simulink model "AEBMIL"  (Simulink 8.2)
settings: Solver=FixedStepDiscrete  StartTime=0.0  StopTime=126  FixedStep=0.005  RelTol=1e-3
PostLoadFcn:
  | , if any(exist('dsrtsu_mdlpostloadfcn', 'file') == [2, 3, 6]), try dsrtsu_mdlpostloadfcn('Execute', bdroot); catch fprintf('Error in PostLoadFcn (dsrtsu_mdlpostloadfcn) for model "%s":\n %s\n', bdroot, lasterr); end, end,
values from neighbouring files (symbols this model uses):
  C_TASK_5MS_S = (	C_TICK_TIME_S      	)    [hcu_local_hdr.m]
  ENUM_GEARPOSN_1ST = uint8(  1  )    [hcu_local_hdr.m]
  ENUM_GEARPOSN_R = uint8(  7  )    [hcu_local_hdr.m]
  FALSE = boolean( 0 )    [hcu_local_hdr.m]
  R_OBJ_Position = single([ii 0 0])    [GridSearch.m]
  R_OBJ_RelAccel = single([0 0 kk])    [GridSearch.m]
  R_OBJ_RelVelocity = single([0 jj 0])    [GridSearch.m]
  TRUE = boolean( 1 )    [hcu_local_hdr.m]
undefined symbols (not defined in the file or in its folder): A_OBJ, AAEB_VehSpd_kph, B_OBJ, C_OBJ, Gamma_OBJ, KAEB_AEBActiveCount_cnt, KAEB_DsblAEBAPPRateThres_pctps, KAEB_DsblAEBSteerRateThres_degps, KAEB_UseMCTTTC_flg, KAEB_VehHoldSpdThres_kph, KOBJ_KalmanFilterCalRate_s, KOBJ_UseCalObjSpd_flg, KOBJ_UseEstObjInfo_flg, KOBJ_VehAccCalRate_s, KOBJ_VehAccFltConst_s, KPTH_ObjPositionYLimit_m, MAEB_AEBTTCThres_s, MAEB_FCWTTCOffset_s, magnitude, MPTH_TurningRadius_m, Q_OBJ, slcm
libraries: simulink x49, hcu_lib x22, dspmtrx3 x3, dspinverses x1
(part 1 of 3)
settings Model: DSRTSU_INTERNAL_RTI_VER=460  DSRTSU_INTERNAL_RTI_TYPE=rti1401  RTICANMMDATA=struct('GeneralSetupData',struct('modelroot','D:\HAITEC\SVN\trunk\ADAS_Softwares\HTDragon\software\sw_development\arch','generalsettings',struct('filesettings',struct('destfolder',struct('Name','RTICANMM_FILES','Check',1),'buildfolder',struct('Name','.','Check',1),'AbsDestfolder',struct('Name','D:\HAITEC\SVN\trunk\ADAS_Softwares\HTDragon\software\sw_development\arch\RTICANMM_FILES'),'AbsBuildfolder',struct('Name','D:\HAITEC\SVN\trunk\ADAS_Softwares\HTDragon\software\sw_development\arch'))),'options',struct('addpaths',1,'rmpaths',1,'addtrcexclusion',logical(1),'cannavigator',struct('checkmonitoring',0),'show_usrtrc',0,'use_usrtrc',0),'advanced',struct('options',[1 1 1 1 1 1 1 1 1 1 1 1 1 1 1 1 1 1 1 1 1 1 1 1 1 1 1 1 1 1 1 1 1 1 1 1 1 1 1 1 1 1 1 1 1 1 1 1 1 1 1 1 1 1 1 1 1 1 1 1 1 1 1 1 1 1 1 1 1 1 1 1 1 1 1 1 1 1 1 1 1 1 1 1 1 1 1 1 1 1 1 1 1 1 1 1 1 1 1 1]),'MPSetup',{{}},'modelname','AEBMIL','block','AEBMIL'))  DSRTSU_INTERNAL_RTIFPGA=50  Creator=14014  LastModifiedBy=14014  BufferReuse=off
settings DataIOCC: SignalLoggingSaveFormat=Dataset
settings OptimizationCC: BlockReduction=off  OptimizeBlockIOStorage=off  BufferReuse=off  ExpressionFolding=off  ExpressionDepthLimit=128  LocalBlockOutputs=off
settings DebuggingCC: FcnCallInpInsideContextMsg=EnableAllAsError  StateNameClashWarn=none
settings HardwareCC: ProdIntDivRoundTo=Zero  ProdEndianess=BigEndian  ProdHWDeviceType=Generic->Custom  TargetIntDivRoundTo=Zero  TargetEndianess=BigEndian  TargetHWDeviceType=Generic->Custom
settings RTWCC: SystemTargetFile=rti1401.tlc  MakeCommand=make_rti  TemplateMakefile=rti1401.tmf  Description=dSPACE DS1401 Hardware Platform  ProcessScript=rti1401_make_rtw_hook
settings STFCustomTargetCC: CodeReplacementLibrary=ANSI_C  ParMdlRefBuildCompliant=on  GeneratePreprocessorConditionals=Disable all  MatFileLogging=on  SystemTargetFile=rti1401.tlc
settings GRTTargetCC: CompOptLevelCompliant=off  ConcurrentExecutionCompliant=off  ExtModeMexFile=noextcomm
settings CustomProperty: DataType=RTWOptions_EnumType_C__Program Files_dSPACE RCPHIL 2015-A_MATLAB_RTI_RTI1401_TLC_rti1401_1InitialSimState  Value=RUN
settings EnumStrPairs: String=RUN

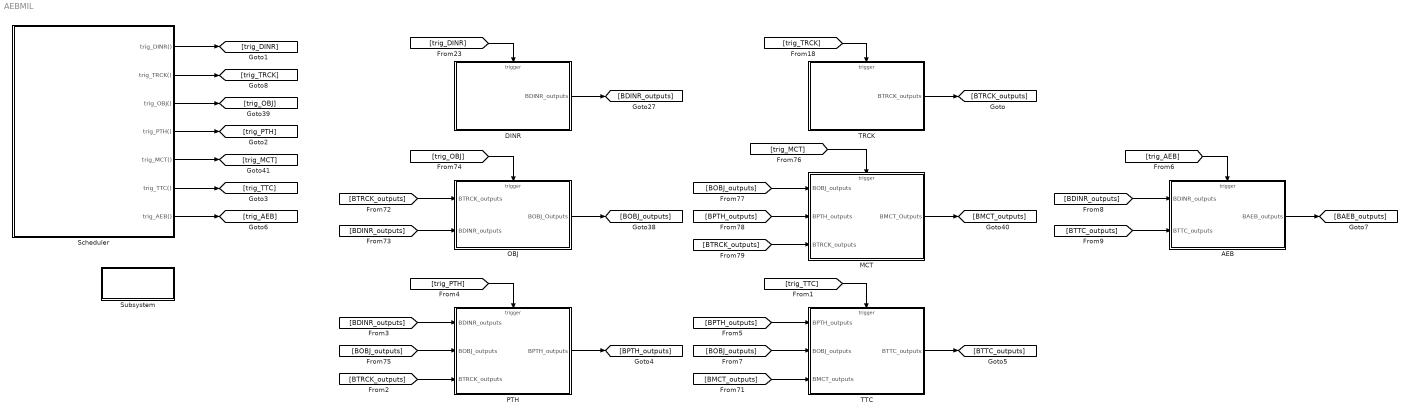
== system AEBMIL ==
  AEB : Subsystem
      settings: RTWSystemCode=Nonreusable function  RTWFcnNameOpts=Use subsystem name  RTWFileNameOpts=Use subsystem name
  DINR : Subsystem
      settings: RTWSystemCode=Nonreusable function  RTWFcnNameOpts=Use subsystem name  RTWFileNameOpts=Use subsystem name
  MCT : Subsystem
      settings: RTWSystemCode=Nonreusable function  RTWFcnNameOpts=Use subsystem name  RTWFileNameOpts=Use subsystem name
  OBJ : Subsystem
      settings: RTWSystemCode=Nonreusable function  RTWFcnNameOpts=Use subsystem name  RTWFileNameOpts=Use subsystem name
  PTH : Subsystem
      settings: RTWSystemCode=Nonreusable function  RTWFcnNameOpts=Use subsystem name  RTWFileNameOpts=Use subsystem name
  Scheduler : Stateflow chart  TreatAsAtomicUnit=on
  Subsystem : Subsystem
      settings: OpenFcn=load AEBMIL_Data.mat;
      mask Display: disp('Double-Click\nTo Load Data')
  TRCK : Subsystem
      settings: RTWSystemCode=Nonreusable function  RTWFcnNameOpts=Use subsystem name  RTWFileNameOpts=Use subsystem name
  TTC : Subsystem
      settings: RTWSystemCode=Nonreusable function  RTWFcnNameOpts=Use subsystem name  RTWFileNameOpts=Use subsystem name
  wires:
  Scheduler/4(trig_PTH()) -> [trig_PTH]
  [BDINR_outputs] -> PTH/1(BDINR_outputs)
  [trig_PTH] -> PTH/Trigger
  PTH/1(BPTH_outputs) -> [BPTH_outputs]
  Scheduler/6(trig_TTC()) -> [trig_TTC]
  [trig_TTC] -> TTC/Trigger
  [BPTH_outputs] -> TTC/1(BPTH_outputs)
  [BOBJ_outputs] -> TTC/2(BOBJ_outputs)
  TTC/1(BTTC_outputs) -> [BTTC_outputs]
  Scheduler/7(trig_AEB()) -> [trig_AEB]
  [trig_AEB] -> AEB/Trigger
  [BDINR_outputs] -> AEB/1(BDINR_outputs)
  [BTTC_outputs] -> AEB/2(BTTC_outputs)
  AEB/1(BAEB_outputs) -> [BAEB_outputs]
  [BMCT_outputs] -> TTC/3(BMCT_outputs)
  [BTRCK_outputs] -> OBJ/1(BTRCK_outputs)
  [BDINR_outputs] -> OBJ/2(BDINR_outputs)
  OBJ/1(BOBJ_Outputs) -> [BOBJ_outputs]
  [trig_OBJ] -> OBJ/Trigger
  Scheduler/3(trig_OBJ()) -> [trig_OBJ]
  [BTRCK_outputs] -> PTH/3(BTRCK_outputs)
  [BOBJ_outputs] -> PTH/2(BOBJ_outputs)
  [trig_MCT] -> MCT/Trigger
  MCT/1(BMCT_Outputs) -> [BMCT_outputs]
  [BOBJ_outputs] -> MCT/1(BOBJ_outputs)
  [BPTH_outputs] -> MCT/2(BPTH_outputs)
  [BTRCK_outputs] -> MCT/3(BTRCK_outputs)
  Scheduler/5(trig_MCT()) -> [trig_MCT]
  [trig_DINR] -> DINR/Trigger
  DINR/1(BDINR_outputs) -> [BDINR_outputs]
  Scheduler/1(trig_DINR()) -> [trig_DINR]
  TRCK/1(BTRCK_outputs) -> [BTRCK_outputs]
  [trig_TRCK] -> TRCK/Trigger
  Scheduler/2(trig_TRCK()) -> [trig_TRCK]

== system AEBMIL/AEB ==
  BDINR_outputs : Inport
  BTTC_outputs : Inport  Port=2  OutDataTypeStr=Bus: BTTC_outputs
  trig_AEB : TriggerPort  TriggerType=function-call
  AEB : Subsystem
  Bus Creator : BusCreator  Inputs=7  OutDataTypeStr=Bus: BAEB_outputs
  Bus Selector : BusSelector  OutputSignals=VTTC_MCTTTC_s,VTTC_Obj1TTCCal_s
  Bus Selector1 : BusSelector  OutputSignals=VDINR_VehSpd_kph,VDINR_SteerAngle_deg,VDINR_SteerAngleValid_flg,VDINR_HWAccelPedalPosn_pct,VDINR_HWAccelPedalPosnValid_flg,VDINR_SeatBeltNOTFasten_flg
  model_info : Subsystem  LoadFcn=slcm LoadBlock;  InitFcn=slcm('UpdateAllCMBlocksInThisModelInit')  mask(CMBlock){InitialSaveTempField=, InitialBlockCM=None, BlockCM=None, Frame=on, SaveTempField=, DisplayStringWithTags=$Id: aeb.mdl 800 2014-08-28 03:32:11Z JuneXmas $, MaskDisplayString=$Id: aeb.mdl 800 2014-08-28 03:32:11Z JuneXmas $, HorizontalTextAlignment=Center, LeftAlignmentValue=0.5, SourceBlockDiagram=AEBMIL, TagMaxNumber=20, CMTag1=, CMTag2=, CMTag3=, CMTag4=, CMTag5=, CMTag6=, CMTag7=, CMTag8=, CMTag9=, CMTag10=, CMTag11=, CMTag12=, CMTag13=, CMTag14=, CMTag15=, CMTag16=, CMTag17=, CMTag18=, CMTag19=, CMTag20=}
      mask help: This block allows revision control information to be displayed within the model.
      settings: CopyFcn=slcm CopyBlock;  DeleteFcn=slcm Cancel;  PostSaveFcn=slcm('UpdateAllCMBlocksInThisModel')  NameChangeFcn=slcm Rename;  OpenFcn=slcm
      mask Display: text(str2num(LeftAlignmentValue), 0.5, MaskDisplayString, 'HorizontalAlignment', HorizontalTextAlignment)
  BAEB_outputs : Outport  OutDataTypeStr=Bus: BAEB_outputs
  wires:
  Bus Selector/2 -> AEB/8(VTTC_Obj1TTCCal_s)  "<VTTC_Obj1TTCCal_s>"
  AEB/7(VAEB_DriverDisable_flg) -> Bus Creator/7
  AEB/6(VAEB_DriverDisableLatch_flg) -> Bus Creator/6
  AEB/5(VAEB_VehHoldReq_flg) -> Bus Creator/5
  AEB/4(VAEB_PreFillReq_flg) -> Bus Creator/4
  AEB/3(VAEB_ForcedIdle_flg) -> Bus Creator/3
  AEB/2(VAEB_FCWActive_flg) -> Bus Creator/2
  AEB/1(VAEB_AEBActive_flg) -> Bus Creator/1
  Bus Creator/1 -> BAEB_outputs/1  "BAEB_outputs"
  BDINR_outputs/1 -> Bus Selector1/1
  Bus Selector1/2 -> AEB/2(VDINR_SteerAngle_deg)  "<VDINR_SteerAngle_deg>"
  Bus Selector1/3 -> AEB/3(VDINR_SteerAngleValid_flg)  "<VDINR_SteerAngleValid_flg>"
  Bus Selector1/4 -> AEB/4(VDINR_HWAccelPedalPosn_pct)  "<VDINR_HWAccelPedalPosn_pct>"
  Bus Selector1/5 -> AEB/5(VDINR_HWAccelPedalPosnValid_flg)  "<VDINR_HWAccelPedalPosnValid_flg>"
  Bus Selector1/6 -> AEB/6(VDINR_SeatBeltNOTFasten_flg)  "<VDINR_SeatBeltNOTFasten_flg>"
  Bus Selector/1 -> AEB/7(VTTC_MCTTTC_s)  "<VTTC_MCTTTC_s>"
  BTTC_outputs/1 -> Bus Selector/1
  Bus Selector1/1 -> AEB/1(VDINR_VehSpd_kph)  "<VDINR_VehSpd_kph>"

== system AEBMIL/DINR ==
  trig_DINR : TriggerPort  TriggerType=function-call
  Bus Creator : BusCreator  Inputs=7
  Cast173 : DataTypeConversion  OutDataTypeStr=boolean  RndMeth=Zero
  Cast202 : DataTypeConversion  OutDataTypeStr=uint8  RndMeth=Zero
  Cast222 : DataTypeConversion  OutDataTypeStr=single  RndMeth=Zero
  Cast259 : DataTypeConversion  OutDataTypeStr=single  RndMeth=Zero
  Cast260 : DataTypeConversion  OutDataTypeStr=boolean  RndMeth=Zero
  Cast89 : DataTypeConversion  OutDataTypeStr=single  RndMeth=Zero
  Cast91 : DataTypeConversion  OutDataTypeStr=boolean  RndMeth=Zero
  Constant : Constant  Value=ENUM_GEARPOSN_1ST
  Constant1 : Constant  Value=TRUE
  Constant2 : Constant  Value=FALSE
  Constant3 : Constant  Value=TRUE
  Constant4 : Constant  Value=single(0)
  From Workspace : FromWorkspace  VariableName=[SimTime VehSpd_kph]
  From Workspace1 : FromWorkspace  VariableName=[SimTime SteerAngle_deg]
  BDINR_outputs : Outport
  wires:
  Constant3/1 -> Cast260/1
  Constant4/1 -> Cast259/1
  Constant2/1 -> Cast173/1
  From Workspace1/1 -> Cast222/1
  Constant1/1 -> Cast91/1
  From Workspace/1 -> Cast89/1
  Constant/1 -> Cast202/1
  Cast260/1 -> Bus Creator/7  "VDINR_HWAccelPedalPosnValid_flg"
  Cast259/1 -> Bus Creator/6  "VDINR_HWAccelPedalPosn_pct"
  Cast173/1 -> Bus Creator/5  "VDINR_SeatBeltNOTFasten_flg"
  Cast202/1 -> Bus Creator/1  "VDINR_NowGearPosn_enum"
  Cast222/1 -> Bus Creator/3  "VDINR_SteerAngle_deg"
  Cast91/1 -> Bus Creator/4  "VDINR_SteerAngleValid_flg"
  Cast89/1 -> Bus Creator/2  "VDINR_VehSpd_kph"
  Bus Creator/1 -> BDINR_outputs/1  "BDINR_outputs"

== system AEBMIL/MCT ==
  BOBJ_outputs : Inport  OutDataTypeStr=Bus: BOBJ_outputs
  BPTH_outputs : Inport  Port=2  OutDataTypeStr=Bus: BPTH_outputs
  BTRCK_outputs : Inport  Port=3  OutDataTypeStr=Bus: BTRCK_outputs
  trig_MCT : TriggerPort  TriggerType=function-call
  Bus Creator : BusCreator  Inputs=5  OutDataTypeStr=Bus: BMCT_outputs
  Bus Selector1 : BusSelector  OutputSignals=VTRCK_Obj1PositionY_m,VTRCK_Obj2PositionY_m,VTRCK_Obj3PositionY_m,VTRCK_Obj4PositionY_m,VTRCK_Obj5PositionY_m
  Bus Selector3 : BusSelector  OutputSignals=VOBJ_Obj1PositionX_m,VOBJ_Obj2PositionX_m,VOBJ_Obj3PositionX_m,VOBJ_Obj4PositionX_m,VOBJ_Obj5PositionX_m,VOBJ_Obj1RelVelocityX_mps,VOBJ_Obj2RelVelocityX_mps,VOBJ_Obj3RelVelocityX_mps,VOBJ_Obj4RelVelocityX_mps,VOBJ_Obj5RelVelocityX_mps,VOBJ_Obj1RelAccX_mps2,VOBJ_Obj2RelAccX_mps2,VOBJ_Obj3RelAccX_mps2,VOBJ_Obj4RelAccX_mps2,VOBJ_Obj5RelAccX_mps2,VOBJ_Obj1Valid_flg,VOBJ_Obj2Valid_flg,VOBJ_Obj3Valid_flg,VOBJ_Obj4Valid_flg,VOBJ_Obj5Valid_flg
  Bus Selector5 : BusSelector  OutputSignals=VPTH_HostPathYOfstWRTObj1_m,VPTH_HostPathYOfstWRTObj2_m,VPTH_HostPathYOfstWRTObj3_m,VPTH_HostPathYOfstWRTObj4_m,VPTH_HostPathYOfstWRTObj5_m,VPTH_Obj1InPath_flg,VPTH_Obj2InPath_flg,VPTH_Obj3InPath_flg,VPTH_Obj4InPath_flg,VPTH_Obj5InPath_flg
  MCT : Subsystem
  model_info : Subsystem  LoadFcn=slcm LoadBlock;  InitFcn=slcm('UpdateAllCMBlocksInThisModelInit')  mask(CMBlock){InitialSaveTempField=, InitialBlockCM=None, BlockCM=None, Frame=on, SaveTempField=, DisplayStringWithTags=$Id: ttc.mdl 800 2014-08-28 03:32:11Z JuneXmas $, MaskDisplayString=$Id: ttc.mdl 800 2014-08-28 03:32:11Z JuneXmas $, HorizontalTextAlignment=Center, LeftAlignmentValue=0.5, SourceBlockDiagram=AEBMIL, TagMaxNumber=20, CMTag1=, CMTag2=, CMTag3=, CMTag4=, CMTag5=, CMTag6=, CMTag7=, CMTag8=, CMTag9=, CMTag10=, CMTag11=, CMTag12=, CMTag13=, CMTag14=, CMTag15=, CMTag16=, CMTag17=, CMTag18=, CMTag19=, CMTag20=}
      mask help: This block allows revision control information to be displayed within the model.
      settings: CopyFcn=slcm CopyBlock;  DeleteFcn=slcm Cancel;  PostSaveFcn=slcm('UpdateAllCMBlocksInThisModel')  NameChangeFcn=slcm Rename;  OpenFcn=slcm
      mask Display: text(str2num(LeftAlignmentValue), 0.5, MaskDisplayString, 'HorizontalAlignment', HorizontalTextAlignment)
  BMCT_Outputs : Outport  OutDataTypeStr=Bus: BMCT_outputs
  wires:
  MCT/5(VMCT_MCTInPath_flg) -> Bus Creator/5
  Bus Selector5/6 -> MCT/31(VPTH_Obj1InPath_flg)  "<VPTH_Obj1InPath_flg>"
  Bus Selector5/7 -> MCT/32(VPTH_Obj2InPath_flg)  "<VPTH_Obj2InPath_flg>"
  Bus Selector5/8 -> MCT/33(VPTH_Obj3InPath_flg)  "<VPTH_Obj3InPath_flg>"
  Bus Selector5/9 -> MCT/34(VPTH_Obj4InPath_flg)  "<VPTH_Obj4InPath_flg>"
  Bus Selector5/10 -> MCT/35(VPTH_Obj5InPath_flg)  "<VPTH_Obj5InPath_flg>"
  MCT/4(VMCT_MCTValid_flg) -> Bus Creator/4
  MCT/3(VMCT_MCTRelAccX_mps2) -> Bus Creator/3
  MCT/2(VMCT_MCTRelVelocityX_mps) -> Bus Creator/2
  MCT/1(VMCT_MCTPositionX_m) -> Bus Creator/1
  Bus Selector5/5 -> MCT/30(VPTH_HostPathYOfstWRTObj5_m)  "<VPTH_HostPathYOfstWRTObj5_m>"
  Bus Selector5/4 -> MCT/29(VPTH_HostPathYOfstWRTObj4_m)  "<VPTH_HostPathYOfstWRTObj4_m>"
  Bus Selector5/3 -> MCT/28(VPTH_HostPathYOfstWRTObj3_m)  "<VPTH_HostPathYOfstWRTObj3_m>"
  Bus Selector5/2 -> MCT/27(VPTH_HostPathYOfstWRTObj2_m)  "<VPTH_HostPathYOfstWRTObj2_m>"
  Bus Selector5/1 -> MCT/26(VPTH_HostPathYOfstWRTObj1_m)  "<VPTH_HostPathYOfstWRTObj1_m>"
  Bus Selector1/5 -> MCT/25(VTRCK_Obj5PositionY_m)  "<VTRCK_Obj5PositionY_m>"
  Bus Selector1/4 -> MCT/24(VTRCK_Obj4PositionY_m)  "<VTRCK_Obj4PositionY_m>"
  Bus Selector1/3 -> MCT/23(VTRCK_Obj3PositionY_m)  "<VTRCK_Obj3PositionY_m>"
  Bus Selector1/2 -> MCT/22(VTRCK_Obj2PositionY_m)  "<VTRCK_Obj2PositionY_m>"
  Bus Selector1/1 -> MCT/21(VTRCK_Obj1PositionY_m)  "<VTRCK_Obj1PositionY_m>"
  BTRCK_outputs/1 -> Bus Selector1/1
  Bus Selector3/20 -> MCT/20(VOBJ_Obj5Valid_flg)  "<VOBJ_Obj5Valid_flg>"
  Bus Selector3/19 -> MCT/19(VOBJ_Obj4Valid_flg)  "<VOBJ_Obj4Valid_flg>"
  Bus Selector3/18 -> MCT/18(VOBJ_Obj3Valid_flg)  "<VOBJ_Obj3Valid_flg>"
  Bus Selector3/17 -> MCT/17(VOBJ_Obj2Valid_flg)  "<VOBJ_Obj2Valid_flg>"
  Bus Selector3/16 -> MCT/16(VOBJ_Obj1Valid_flg)  "<VOBJ_Obj1Valid_flg>"
  Bus Selector3/15 -> MCT/15(VOBJ_Obj5RelAccX_mps2)  "<VOBJ_Obj5RelAccX_mps2>"
  Bus Selector3/14 -> MCT/14(VOBJ_Obj4RelAccX_mps2)  "<VOBJ_Obj4RelAccX_mps2>"
  Bus Selector3/13 -> MCT/13(VOBJ_Obj3RelAccX_mps2)  "<VOBJ_Obj3RelAccX_mps2>"
  Bus Selector3/12 -> MCT/12(VOBJ_Obj2RelAccX_mps2)  "<VOBJ_Obj2RelAccX_mps2>"
  Bus Selector3/11 -> MCT/11(VOBJ_Obj1RelAccX_mps2)  "<VOBJ_Obj1RelAccX_mps2>"
  Bus Selector3/10 -> MCT/10(VOBJ_Obj5RelVelocityX_mps)  "<VOBJ_Obj5RelVelocityX_mps>"
  Bus Selector3/9 -> MCT/9(VOBJ_Obj4RelVelocityX_mps)  "<VOBJ_Obj4RelVelocityX_mps>"
  Bus Selector3/8 -> MCT/8(VOBJ_Obj3RelVelocityX_mps)  "<VOBJ_Obj3RelVelocityX_mps>"
  Bus Selector3/7 -> MCT/7(VOBJ_Obj2RelVelocityX_mps)  "<VOBJ_Obj2RelVelocityX_mps>"
  Bus Selector3/6 -> MCT/6(VOBJ_Obj1RelVelocityX_mps)  "<VOBJ_Obj1RelVelocityX_mps>"
  Bus Selector3/5 -> MCT/5(VObj_Obj5PositionX_m)  "<VOBJ_Obj5PositionX_m>"
  Bus Selector3/1 -> MCT/1(VOBJ_Obj1PositionX_m)  "<VOBJ_Obj1PositionX_m>"
  Bus Selector3/4 -> MCT/4(VOBJ_Obj4PositionX_m)  "<VOBJ_Obj4PositionX_m>"
  Bus Selector3/2 -> MCT/2(VOBJ_Obj2PositionX_m)  "<VOBJ_Obj2PositionX_m>"
  Bus Selector3/3 -> MCT/3(VOBJ_Obj3PositionX_m)  "<VOBJ_Obj3PositionX_m>"
  BPTH_outputs/1 -> Bus Selector5/1
  BOBJ_outputs/1 -> Bus Selector3/1
  Bus Creator/1 -> BMCT_Outputs/1  "BMCT_outputs"

== system AEBMIL/OBJ ==
  BTRCK_outputs : Inport  OutDataTypeStr=Bus: BTRCK_outputs
  BDINR_outputs : Inport  Port=2
  trig_OBJ : TriggerPort  TriggerType=function-call
  Bus Creator : BusCreator  Inputs=20  OutDataTypeStr=Bus: BOBJ_outputs
  Bus Selector3 : BusSelector  OutputSignals=VTRCK_Obj1PositionX_m,VTRCK_Obj1RelVelocityX_mps,VTRCK_Obj1Valid_flg,VTRCK_Obj1ConfidLevel_enum,VTRCK_Obj2PositionX_m,VTRCK_Obj2RelVelocityX_mps,VTRCK_Obj2Valid_flg,VTRCK_Obj2ConfidLevel_enum,VTRCK_Obj3PositionX_m,VTRCK_Obj3RelVelocityX_mps,VTRCK_Obj3Valid_flg,VTRCK_Obj3ConfidLevel_enum,VTRCK_Obj4PositionX_m,VTRCK_Obj4RelVelocityX_mps,VTRCK_Obj4Valid_flg,VTRCK_Obj4ConfidLevel_enum,VTRCK_Obj5PositionX_m,VTRCK_Obj5RelVelocityX_mps,VTRCK_Obj5Valid_flg,VTRCK_Obj5ConfidLevel_enum
  Bus Selector5 : BusSelector  OutputSignals=VDINR_VehSpd_kph,VDINR_NowGearPosn_enum
  OBJ : Subsystem
  model_info : Subsystem  LoadFcn=slcm LoadBlock;  InitFcn=slcm('UpdateAllCMBlocksInThisModelInit')  mask(CMBlock){InitialSaveTempField=, InitialBlockCM=None, BlockCM=None, Frame=on, SaveTempField=, DisplayStringWithTags=$Id: ttc.mdl 800 2014-08-28 03:32:11Z JuneXmas $, MaskDisplayString=$Id: ttc.mdl 800 2014-08-28 03:32:11Z JuneXmas $, HorizontalTextAlignment=Center, LeftAlignmentValue=0.5, SourceBlockDiagram=AEBMIL, TagMaxNumber=20, CMTag1=, CMTag2=, CMTag3=, CMTag4=, CMTag5=, CMTag6=, CMTag7=, CMTag8=, CMTag9=, CMTag10=, CMTag11=, CMTag12=, CMTag13=, CMTag14=, CMTag15=, CMTag16=, CMTag17=, CMTag18=, CMTag19=, CMTag20=}
      mask help: This block allows revision control information to be displayed within the model.
      settings: CopyFcn=slcm CopyBlock;  DeleteFcn=slcm Cancel;  PostSaveFcn=slcm('UpdateAllCMBlocksInThisModel')  NameChangeFcn=slcm Rename;  OpenFcn=slcm
      mask Display: text(str2num(LeftAlignmentValue), 0.5, MaskDisplayString, 'HorizontalAlignment', HorizontalTextAlignment)
  BOBJ_Outputs : Outport  OutDataTypeStr=Bus: BOBJ_outputs
  wires:
  Bus Creator/1 -> BOBJ_Outputs/1  "BOBJ_outputs"
  BTRCK_outputs/1 -> Bus Selector3/1
  Bus Selector3/14 -> OBJ/14(VTRCK_Obj4RelVelocityX_mps)  "<VTRCK_Obj4RelVelocityX_mps>"
  Bus Selector3/10 -> OBJ/10(VTRCK_Obj3RelVelocityX_mps)  "<VTRCK_Obj3RelVelocityX_mps>"
  Bus Selector3/9 -> OBJ/9(VTRCK_Obj3PositionX_m)  "<VTRCK_Obj3PositionX_m>"
  Bus Selector3/2 -> OBJ/2(VTRCK_Obj1RelVelocityX_mps)  "<VTRCK_Obj1RelVelocityX_mps>"
  Bus Selector3/6 -> OBJ/6(VTRCK_Obj2RelVelocityX_mps)  "<VTRCK_Obj2RelVelocityX_mps>"
  Bus Selector3/18 -> OBJ/18(VTRCK_Obj5RelVelocityX_mps)  "<VTRCK_Obj5RelVelocityX_mps>"
  Bus Selector3/1 -> OBJ/1(VTRCK_Obj1PositionX_m)  "<VTRCK_Obj1PositionX_m>"
  Bus Selector3/5 -> OBJ/5(VTRCK_Obj2PositionX_m)  "<VTRCK_Obj2PositionX_m>"
  Bus Selector3/13 -> OBJ/13(VTRCK_Obj4PositionX_m)  "<VTRCK_Obj4PositionX_m>"
  Bus Selector3/17 -> OBJ/17(VTRCK_Obj5PositionX_m)  "<VTRCK_Obj5PositionX_m>"
  Bus Selector5/1 -> OBJ/21(VDINR_VehSpd_kph)  "<VDINR_VehSpd_kph>"
  BDINR_outputs/1 -> Bus Selector5/1
  Bus Selector3/3 -> OBJ/3(VTRCK_Obj1Valid_flg)  "<VTRCK_Obj1Valid_flg>"
  Bus Selector3/7 -> OBJ/7(VTRCK_Obj2Valid_flg)  "<VTRCK_Obj2Valid_flg>"
  Bus Selector3/11 -> OBJ/11(VTRCK_Obj3Valid_flg)  "<VTRCK_Obj3Valid_flg>"
  Bus Selector3/15 -> OBJ/15(VTRCK_Obj4Valid_flg)  "<VTRCK_Obj4Valid_flg>"
  Bus Selector3/19 -> OBJ/19(VTRCK_Obj5Valid_flg)  "<VTRCK_Obj5Valid_flg>"
  OBJ/1(VOBJ_Obj1PositionX_m) -> Bus Creator/1
  OBJ/2(VOBJ_Obj1RelVelocityX_mps) -> Bus Creator/2
  OBJ/3(VOBJ_Obj1RelAccX_mps2) -> Bus Creator/3
  OBJ/4(VOBJ_Obj1Valid_flg) -> Bus Creator/4
  OBJ/5(VOBJ_Obj2PositionX_m) -> Bus Creator/5
  OBJ/6(VOBJ_Obj2RelVelocityX_mps) -> Bus Creator/6
  OBJ/7(VOBJ_Obj2RelAccX_mps2) -> Bus Creator/7
  OBJ/8(VOBJ_Obj2Valid_flg) -> Bus Creator/8
  OBJ/9(VOBJ_Obj3PositionX_m) -> Bus Creator/9
  OBJ/10(VOBJ_Obj3RelVelocityX_mps) -> Bus Creator/10
  OBJ/11(VOBJ_Obj3RelAccX_mps2) -> Bus Creator/11
  OBJ/12(VOBJ_Obj3Valid_flg) -> Bus Creator/12
  OBJ/13(VOBJ_Obj4PositionX_m) -> Bus Creator/13
  OBJ/14(VOBJ_Obj4RelVelocityX_mps) -> Bus Creator/14
  OBJ/15(VOBJ_Obj4RelAccX_mps2) -> Bus Creator/15
  OBJ/16(VOBJ_Obj4Valid_flg) -> Bus Creator/16
  OBJ/17(VOBJ_Obj5PositionX_m) -> Bus Creator/17
  OBJ/18(VOBJ_Obj5RelVelocityX_mps) -> Bus Creator/18
  OBJ/19(VOBJ_Obj5RelAccX_mps2) -> Bus Creator/19
  OBJ/20(VOBJ_Obj5Valid_flg) -> Bus Creator/20
  Bus Selector5/2 -> OBJ/22(VDINR_NowGearPosn_enum)  "<VDINR_NowGearPosn_enum>"
  Bus Selector3/4 -> OBJ/4(VTRCK_Obj1ConfidLevel_enum)  "<VTRCK_Obj1ConfidLevel_enum>"
  Bus Selector3/8 -> OBJ/8(VTRCK_Obj2ConfidLevel_enum)  "<VTRCK_Obj2ConfidLevel_enum>"
  Bus Selector3/12 -> OBJ/12(VTRCK_Obj3ConfidLevel_enum)  "<VTRCK_Obj3ConfidLevel_enum>"
  Bus Selector3/16 -> OBJ/16(VTRCK_Obj4ConfidLevel_enum)  "<VTRCK_Obj4ConfidLevel_enum>"
  Bus Selector3/20 -> OBJ/20(VTRCK_Obj5ConfidLevel_enum)  "<VTRCK_Obj5ConfidLevel_enum>"

== system AEBMIL/PTH ==
  BDINR_outputs : Inport
  BOBJ_outputs : Inport  Port=2  OutDataTypeStr=Bus: BOBJ_outputs
  BTRCK_outputs : Inport  Port=3  OutDataTypeStr=Bus: BTRCK_outputs
  trig_PTH : TriggerPort  TriggerType=function-call
  Bus Creator : BusCreator  Inputs=10  OutDataTypeStr=Bus: BPTH_outputs
  Bus Selector : BusSelector  OutputSignals=VDINR_VehSpd_kph,VDINR_SteerAngle_deg,VDINR_SteerAngleValid_flg
  Bus Selector1 : BusSelector  OutputSignals=VTRCK_Obj1PositionY_m,VTRCK_Obj2PositionY_m,VTRCK_Obj3PositionY_m,VTRCK_Obj4PositionY_m,VTRCK_Obj5PositionY_m
  Bus Selector2 : BusSelector  OutputSignals=VOBJ_Obj1PositionX_m,VOBJ_Obj2PositionX_m,VOBJ_Obj3PositionX_m,VOBJ_Obj4PositionX_m,VOBJ_Obj5PositionX_m,VOBJ_Obj1Valid_flg,VOBJ_Obj2Valid_flg,VOBJ_Obj3Valid_flg,VOBJ_Obj4Valid_flg,VOBJ_Obj5Valid_flg
  PathEstimation : Subsystem
  model_info : Subsystem  LoadFcn=slcm LoadBlock;  InitFcn=slcm('UpdateAllCMBlocksInThisModelInit')  mask(CMBlock){InitialSaveTempField=, InitialBlockCM=None, BlockCM=None, Frame=on, SaveTempField=, DisplayStringWithTags=$Id: pth.mdl 800 2014-08-28 03:32:11Z JuneXmas $, MaskDisplayString=$Id: pth.mdl 800 2014-08-28 03:32:11Z JuneXmas $, HorizontalTextAlignment=Center, LeftAlignmentValue=0.5, SourceBlockDiagram=AEBMIL, TagMaxNumber=20, CMTag1=, CMTag2=, CMTag3=, CMTag4=, CMTag5=, CMTag6=, CMTag7=, CMTag8=, CMTag9=, CMTag10=, CMTag11=, CMTag12=, CMTag13=, CMTag14=, CMTag15=, CMTag16=, CMTag17=, CMTag18=, CMTag19=, CMTag20=}
      mask help: This block allows revision control information to be displayed within the model.
      settings: CopyFcn=slcm CopyBlock;  DeleteFcn=slcm Cancel;  PostSaveFcn=slcm('UpdateAllCMBlocksInThisModel')  NameChangeFcn=slcm Rename;  OpenFcn=slcm
      mask Display: text(str2num(LeftAlignmentValue), 0.5, MaskDisplayString, 'HorizontalAlignment', HorizontalTextAlignment)
  BPTH_outputs : Outport  OutDataTypeStr=Bus: BPTH_outputs
  wires:
  PathEstimation/10(VPTH_HostPathYOfstWRTObj5_m) -> Bus Creator/10
  PathEstimation/9(VPTH_HostPathYOfstWRTObj4_m) -> Bus Creator/9
  PathEstimation/8(VPTH_HostPathYOfstWRTObj3_m) -> Bus Creator/8
  PathEstimation/7(VPTH_HostPathYOfstWRTObj2_m) -> Bus Creator/7
  PathEstimation/6(VPTH_HostPathYOfstWRTObj1_m) -> Bus Creator/6
  Bus Selector2/7 -> PathEstimation/10(VOBJ_Obj2Valid_flg)  "<VOBJ_Obj2Valid_flg>"
  Bus Selector2/8 -> PathEstimation/11(VOBJ_Obj3Valid_flg)  "<VOBJ_Obj3Valid_flg>"
  Bus Selector2/6 -> PathEstimation/9(VOBJ_Obj1Valid_flg)  "<VOBJ_Obj1Valid_flg>"
  Bus Selector2/10 -> PathEstimation/13(VOBJ_Obj5Valid_flg)  "<VOBJ_Obj5Valid_flg>"
  Bus Selector2/9 -> PathEstimation/12(VOBJ_Obj4Valid_flg)  "<VOBJ_Obj4Valid_flg>"
  Bus Selector2/4 -> PathEstimation/7(VOBJ_Obj4PositionX_m)  "<VOBJ_Obj4PositionX_m>"
  Bus Selector2/2 -> PathEstimation/5(VOBJ_Obj2PositionX_m)  "<VOBJ_Obj2PositionX_m>"
  Bus Selector2/5 -> PathEstimation/8(VOBJ_Obj5PositionX_m)  "<VOBJ_Obj5PositionX_m>"
  Bus Selector2/1 -> PathEstimation/4(VOBJ_Obj1PositionX_m)  "<VOBJ_Obj1PositionX_m>"
  Bus Selector2/3 -> PathEstimation/6(VOBJ_Obj3PositionX_m)  "<VOBJ_Obj3PositionX_m>"
  BOBJ_outputs/1 -> Bus Selector2/1
  PathEstimation/4(VPTH_Obj4InPath_flg) -> Bus Creator/4
  PathEstimation/5(VPTH_Obj5InPath_flg) -> Bus Creator/5
  PathEstimation/2(VPTH_Obj2InPath_flg) -> Bus Creator/2
  PathEstimation/1(VPTH_Obj1InPath_flg) -> Bus Creator/1
  PathEstimation/3(VPTH_Obj3InPath_flg) -> Bus Creator/3
  Bus Selector1/5 -> PathEstimation/18(VTRCK_Obj5PositionY_m)  "<VTRCK_Obj5PositionY_m>"
  Bus Selector1/4 -> PathEstimation/17(VTRCK_Obj4PositionY_m)  "<VTRCK_Obj4PositionY_m>"
  Bus Selector1/3 -> PathEstimation/16(VTRCK_Obj3PositionY_m)  "<VTRCK_Obj3PositionY_m>"
  Bus Selector1/2 -> PathEstimation/15(VTRCK_Obj2PositionY_m)  "<VTRCK_Obj2PositionY_m>"
  Bus Selector1/1 -> PathEstimation/14(VTRCK_Obj1PositionY_m)  "<VTRCK_Obj1PositionY_m>"
  BDINR_outputs/1 -> Bus Selector/1
  Bus Creator/1 -> BPTH_outputs/1  "BPTH_outputs"
  Bus Selector/2 -> PathEstimation/2(VDINR_SteerAngle_deg)  "<VDINR_SteerAngle_deg>"
  BTRCK_outputs/1 -> Bus Selector1/1
  Bus Selector/3 -> PathEstimation/3(VDINR_SteerAngleValid_flg)  "<VDINR_SteerAngleValid_flg>"
  Bus Selector/1 -> PathEstimation/1(VDINR_VehSpd_kph)  "<VDINR_VehSpd_kph>"

== system AEBMIL/Subsystem ==

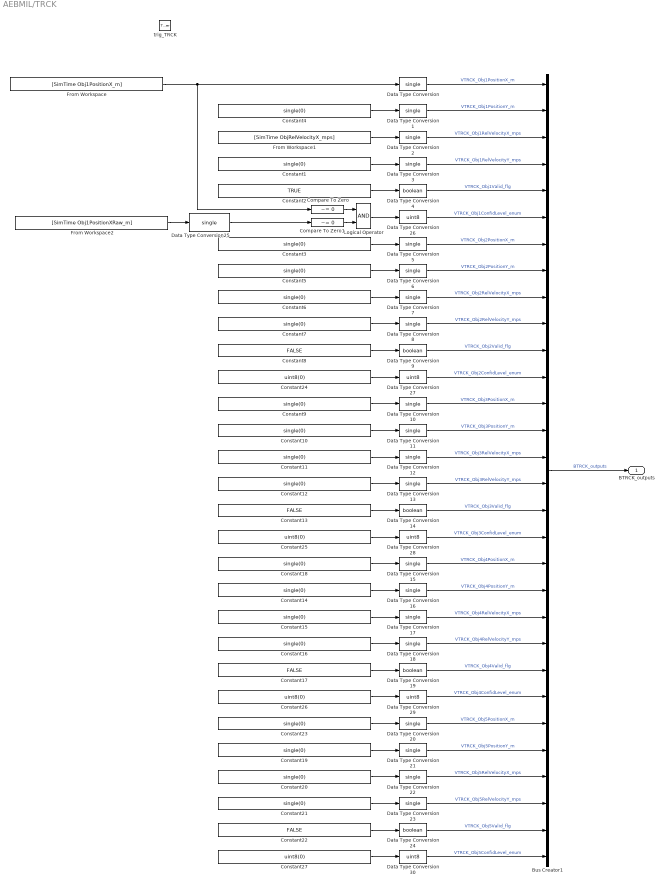
== system AEBMIL/TRCK ==
  trig_TRCK : TriggerPort  TriggerType=function-call
  Bus Creator1 : BusCreator  Inputs=30  OutDataTypeStr=Bus: BTRCK_outputs
  Compare To Zero : simulink/Logic and Bit Operations/Compare To Zero  relop=~=  OutDataTypeStr=boolean
  Compare To Zero1 : simulink/Logic and Bit Operations/Compare To Zero  relop=~=  OutDataTypeStr=boolean
  Constant{1,3..7,9..12,14..16,18..21,23} (18 alike) : Constant  Value=single(0)
  Constant{8,13,17,22} (4 alike) : Constant  Value=FALSE
  Constant2 : Constant  Value=TRUE
  Constant{24..27} (4 alike) : Constant  Value=uint8(0)
  Data Type Conversion{,1..3,5..8,10..13,15..18,20..23,25} (21 alike) : DataTypeConversion  OutDataTypeStr=single
  Data Type Conversion{4,9,14,19,24} (5 alike) : DataTypeConversion  OutDataTypeStr=boolean
  Data Type Conversion{26..30} (5 alike) : DataTypeConversion  OutDataTypeStr=uint8
  From Workspace : FromWorkspace  VariableName=[SimTime Obj1PositionX_m]  Interpolate=off  OutputAfterFinalValue=Setting to zero
  From Workspace1 : FromWorkspace  VariableName=[SimTime ObjRelVelocityX_mps]  Interpolate=off  OutputAfterFinalValue=Setting to zero
  From Workspace2 : FromWorkspace  VariableName=[SimTime Obj1PositionXRaw_m]  Interpolate=off  OutputAfterFinalValue=Setting to zero
  Logical Operator : Logic  AllPortsSameDT=off  OutDataTypeStr=boolean
  BTRCK_outputs : Outport  OutDataTypeStr=Bus: BTRCK_outputs
  wires:
  Bus Creator1/1 -> BTRCK_outputs/1  "BTRCK_outputs"
  Constant4/1 -> Data Type Conversion1/1
  From Workspace1/1 -> Data Type Conversion2/1
  Constant1/1 -> Data Type Conversion3/1
  Constant3/1 -> Data Type Conversion5/1
  Constant5/1 -> Data Type Conversion6/1
  Constant6/1 -> Data Type Conversion7/1
  Constant7/1 -> Data Type Conversion8/1
  Constant9/1 -> Data Type Conversion10/1
  Constant10/1 -> Data Type Conversion11/1
  Constant11/1 -> Data Type Conversion12/1
  Constant12/1 -> Data Type Conversion13/1
  Constant18/1 -> Data Type Conversion15/1
  Constant14/1 -> Data Type Conversion16/1
  Constant15/1 -> Data Type Conversion17/1
  Constant16/1 -> Data Type Conversion18/1
  Constant23/1 -> Data Type Conversion20/1
  Constant19/1 -> Data Type Conversion21/1
  Constant20/1 -> Data Type Conversion22/1
  Constant21/1 -> Data Type Conversion23/1
  Data Type Conversion3/1 -> Bus Creator1/4  "VTRCK_Obj1RelVelocityY_mps"
  Data Type Conversion1/1 -> Bus Creator1/2  "VTRCK_Obj1PositionY_m"
  Data Type Conversion2/1 -> Bus Creator1/3  "VTRCK_Obj1RelVelocityX_mps"
  Data Type Conversion/1 -> Bus Creator1/1  "VTRCK_Obj1PositionX_m"
  Data Type Conversion15/1 -> Bus Creator1/19  "VTRCK_Obj4PositionX_m"
  Data Type Conversion18/1 -> Bus Creator1/22  "VTRCK_Obj4RelVelocityY_mps"
  Data Type Conversion17/1 -> Bus Creator1/21  "VTRCK_Obj4RelVelocityX_mps"
  Data Type Conversion16/1 -> Bus Creator1/20  "VTRCK_Obj4PositionY_m"
  Data Type Conversion22/1 -> Bus Creator1/27  "VTRCK_Obj5RelVelocityX_mps"
  Data Type Conversion19/1 -> Bus Creator1/23  "VTRCK_Obj4Valid_flg"
  Data Type Conversion4/1 -> Bus Creator1/5  "VTRCK_Obj1Valid_flg"
  Data Type Conversion8/1 -> Bus Creator1/10  "VTRCK_Obj2RelVelocityY_mps"
  Data Type Conversion5/1 -> Bus Creator1/7  "VTRCK_Obj2PositionX_m"
  Data Type Conversion6/1 -> Bus Creator1/8  "VTRCK_Obj2PositionY_m"
  Data Type Conversion9/1 -> Bus Creator1/11  "VTRCK_Obj2Valid_flg"
  Data Type Conversion7/1 -> Bus Creator1/9  "VTRCK_Obj2RelVelocityX_mps"
  Data Type Conversion11/1 -> Bus Creator1/14  "VTRCK_Obj3PositionY_m"
  Data Type Conversion12/1 -> Bus Creator1/15  "VTRCK_Obj3RelVelocityX_mps"
  Data Type Conversion13/1 -> Bus Creator1/16  "VTRCK_Obj3RelVelocityY_mps"
  Data Type Conversion14/1 -> Bus Creator1/17  "VTRCK_Obj3Valid_flg"
  Data Type Conversion10/1 -> Bus Creator1/13  "VTRCK_Obj3PositionX_m"
  Data Type Conversion20/1 -> Bus Creator1/25  "VTRCK_Obj5PositionX_m"
  Data Type Conversion21/1 -> Bus Creator1/26  "VTRCK_Obj5PositionY_m"
  Data Type Conversion24/1 -> Bus Creator1/29  "VTRCK_Obj5Valid_flg"
  Data Type Conversion23/1 -> Bus Creator1/28  "VTRCK_Obj5RelVelocityY_mps"
  Constant2/1 -> Data Type Conversion4/1
  Constant8/1 -> Data Type Conversion9/1
  Constant13/1 -> Data Type Conversion14/1
  Constant17/1 -> Data Type Conversion19/1
  Constant22/1 -> Data Type Conversion24/1
  Logical Operator/1 -> Data Type Conversion26/1
  Data Type Conversion26/1 -> Bus Creator1/6  "VTRCK_Obj1ConfidLevel_enum"
  Data Type Conversion27/1 -> Bus Creator1/12  "VTRCK_Obj2ConfidLevel_enum"
  Constant24/1 -> Data Type Conversion27/1
  Data Type Conversion28/1 -> Bus Creator1/18  "VTRCK_Obj3ConfidLevel_enum"
  Constant25/1 -> Data Type Conversion28/1
  Data Type Conversion29/1 -> Bus Creator1/24  "VTRCK_Obj4ConfidLevel_enum"
  Constant26/1 -> Data Type Conversion29/1
  Data Type Conversion30/1 -> Bus Creator1/30  "VTRCK_Obj5ConfidLevel_enum"
  Constant27/1 -> Data Type Conversion30/1
  Compare To Zero1/1 -> Logical Operator/2
  Compare To Zero/1 -> Logical Operator/1
  Data Type Conversion25/1 -> Compare To Zero1/1
  From Workspace2/1 -> Data Type Conversion25/1
  From Workspace/1 -> Compare To Zero/1, Data Type Conversion/1

== system AEBMIL/TTC ==
  BPTH_outputs : Inport  OutDataTypeStr=Bus: BPTH_outputs
  BOBJ_outputs : Inport  Port=2  OutDataTypeStr=Bus: BOBJ_outputs
  BMCT_outputs : Inport  Port=3  OutDataTypeStr=Bus: BMCT_outputs
  trig_TTC : TriggerPort  TriggerType=function-call
  Bus Creator : BusCreator  Inputs=6  OutDataTypeStr=Bus: BTTC_outputs
  Bus Selector2 : BusSelector  OutputSignals=VPTH_Obj1InPath_flg,VPTH_Obj2InPath_flg,VPTH_Obj3InPath_flg,VPTH_Obj4InPath_flg,VPTH_Obj5InPath_flg
  Bus Selector3 : BusSelector  OutputSignals=VOBJ_Obj1PositionX_m,VOBJ_Obj1RelVelocityX_mps,VOBJ_Obj2PositionX_m,VOBJ_Obj2RelVelocityX_mps,VOBJ_Obj3PositionX_m,VOBJ_Obj3RelVelocityX_mps,VOBJ_Obj4PositionX_m,VOBJ_Obj4RelVelocityX_mps,VOBJ_Obj5PositionX_m,VOBJ_Obj5RelVelocityX_mps
  Bus Selector4 : BusSelector  OutputSignals=VMCT_MCTPositionX_m,VMCT_MCTRelVelocityX_mps,VMCT_MCTValid_flg,VMCT_MCTInPath_flg
  MCT_TTC_Calculation : Subsystem
  Mux : Mux  Inputs=2
  Scope2 : Scope
      settings: SaveName=ScopeData17
  TimeToCollisionCal : Subsystem
  model_info : Subsystem  LoadFcn=slcm LoadBlock;  InitFcn=slcm('UpdateAllCMBlocksInThisModelInit')  mask(CMBlock){InitialSaveTempField=, InitialBlockCM=None, BlockCM=None, Frame=on, SaveTempField=, DisplayStringWithTags=$Id: ttc.mdl 800 2014-08-28 03:32:11Z JuneXmas $, MaskDisplayString=$Id: ttc.mdl 800 2014-08-28 03:32:11Z JuneXmas $, HorizontalTextAlignment=Center, LeftAlignmentValue=0.5, SourceBlockDiagram=AEBMIL, TagMaxNumber=20, CMTag1=, CMTag2=, CMTag3=, CMTag4=, CMTag5=, CMTag6=, CMTag7=, CMTag8=, CMTag9=, CMTag10=, CMTag11=, CMTag12=, CMTag13=, CMTag14=, CMTag15=, CMTag16=, CMTag17=, CMTag18=, CMTag19=, CMTag20=}
      mask help: This block allows revision control information to be displayed within the model.
      settings: CopyFcn=slcm CopyBlock;  DeleteFcn=slcm Cancel;  PostSaveFcn=slcm('UpdateAllCMBlocksInThisModel')  NameChangeFcn=slcm Rename;  OpenFcn=slcm
      mask Display: text(str2num(LeftAlignmentValue), 0.5, MaskDisplayString, 'HorizontalAlignment', HorizontalTextAlignment)
  BTTC_outputs : Outport  OutDataTypeStr=Bus: BTTC_outputs
  wires:
  Bus Selector4/4 -> MCT_TTC_Calculation/4(VMCT_MCTInPath_flg)  "<VMCT_MCTInPath_flg>"
  Bus Selector4/3 -> MCT_TTC_Calculation/3(VMCT_MCTValid_flg)  "<VMCT_MCTValid_flg>"
  Bus Selector4/2 -> MCT_TTC_Calculation/2(VMCT_MCTRelVelocityX_mps)  "<VMCT_MCTRelVelocityX_mps>"
  Bus Selector4/1 -> MCT_TTC_Calculation/1(VMCT_MCTRelPositionX_m)  "<VMCT_MCTPositionX_m>"
  MCT_TTC_Calculation/1(VTTC_MCTTTC_s) -> Mux/2, Bus Creator/6
  TimeToCollisionCal/2(VTTC_Obj2TTCCal_s) -> Bus Creator/2
  TimeToCollisionCal/3(VTTC_Obj3TTCCal_s) -> Bus Creator/3
  TimeToCollisionCal/5(VTTC_Obj5TTCCal_s) -> Bus Creator/5
  TimeToCollisionCal/4(VTTC_Obj4TTCCal_s) -> Bus Creator/4
  TimeToCollisionCal/1(VTTC_Obj1TTCCal_s) -> Mux/1, Bus Creator/1
  BMCT_outputs/1 -> Bus Selector4/1
  Bus Selector3/9 -> TimeToCollisionCal/9(VOBJ_Obj5PositionX_m)  "<VOBJ_Obj5PositionX_m>"
  Bus Selector3/7 -> TimeToCollisionCal/7(VOBJ_Obj4PositionX_m)  "<VOBJ_Obj4PositionX_m>"
  Bus Selector3/3 -> TimeToCollisionCal/3(VOBJ_Obj2PositionX_m)  "<VOBJ_Obj2PositionX_m>"
  Bus Selector3/1 -> TimeToCollisionCal/1(VOBJ_Obj1PositionX_m)  "<VOBJ_Obj1PositionX_m>"
  Bus Selector3/10 -> TimeToCollisionCal/10(VOBJ_Obj5RelVelocityX_mps)  "<VOBJ_Obj5RelVelocityX_mps>"
  Bus Selector3/4 -> TimeToCollisionCal/4(VOBJ_Obj2RelVelocityX_mps)  "<VOBJ_Obj2RelVelocityX_mps>"
  Bus Selector3/2 -> TimeToCollisionCal/2(VOBJ_Obj1RelVelocityX_mps)  "<VOBJ_Obj1RelVelocityX_mps>"
  Bus Selector3/5 -> TimeToCollisionCal/5(VOBJ_Obj3PositionX_m)  "<VOBJ_Obj3PositionX_m>"
  Bus Selector3/6 -> TimeToCollisionCal/6(VOBJ_Obj3RelVelocityX_mps)  "<VOBJ_Obj3RelVelocityX_mps>"
  Bus Selector3/8 -> TimeToCollisionCal/8(VOBJ_Obj4RelVelocityX_mps)  "<VOBJ_Obj4RelVelocityX_mps>"
  Bus Selector2/5 -> TimeToCollisionCal/15(VPTH_Obj5InPath_flg)  "<VPTH_Obj5InPath_flg>"
  Bus Selector2/4 -> TimeToCollisionCal/14(VPTH_Obj4InPath_flg)  "<VPTH_Obj4InPath_flg>"
  Bus Selector2/3 -> TimeToCollisionCal/13(VPTH_Obj3InPath_flg)  "<VPTH_Obj3InPath_flg>"
  Bus Selector2/2 -> TimeToCollisionCal/12(VPTH_Obj2InPath_flg)  "<VPTH_Obj2InPath_flg>"
  Bus Selector2/1 -> TimeToCollisionCal/11(VPTH_Obj1InPath_flg)  "<VPTH_Obj1InPath_flg>"
  BOBJ_outputs/1 -> Bus Selector3/1
  Bus Creator/1 -> BTTC_outputs/1  "BTTC_outputs"
  BPTH_outputs/1 -> Bus Selector2/1
  Mux/1 -> Scope2/1

== system AEBMIL/AEB/AEB ==
  VDINR_VehSpd_kph : Inport
  VDINR_SteerAngle_deg : Inport  Port=2
  VDINR_SteerAngleValid_flg : Inport  Port=3
  VDINR_HWAccelPedalPosn_pct : Inport  Port=4
  VDINR_HWAccelPedalPosnValid_flg : Inport  Port=5
  VDINR_SeatBeltNOTFasten_flg : Inport  Port=6
  VTTC_MCTTTC_s : Inport  Port=7
  VTTC_Obj1TTCCal_s : Inport  Port=8
  AEB Determination : Subsystem
  Driver Disable : Subsystem
  Unit Delay : UnitDelay  SampleTime=-1
  VAEB_AEBActive_flg : Outport
  VAEB_FCWActive_flg : Outport  Port=2
  VAEB_ForcedIdle_flg : Outport  Port=3
  VAEB_PreFillReq_flg : Outport  Port=4
  VAEB_VehHoldReq_flg : Outport  Port=5
  VAEB_DriverDisableLatch_flg : Outport  Port=6
  VAEB_DriverDisable_flg : Outport  Port=7
  wires:
  VTTC_Obj1TTCCal_s/1 -> AEB Determination/6(VTTC_Obj1TTCCal_s)
  Unit Delay/1 -> Driver Disable/5(VAEB_AEBActive_flg)
  [VAEB_AEBActive_flg] -> Unit Delay/1
  AEB Determination/5(VAEB_VehHoldReq_flg) -> VAEB_VehHoldReq_flg/1
  AEB Determination/4(VAEB_PreFillReq_flg) -> VAEB_PreFillReq_flg/1
  VTTC_MCTTTC_s/1 -> AEB Determination/5(VTTC_MCTTTC_s)
  VDINR_SeatBeltNOTFasten_flg/1 -> AEB Determination/3(VDINR_SeatBeltNOTFasten_flg)
  Driver Disable/2(VAEB_DriverDisableLatch_flg) -> AEB Determination/2(VAEB_DriverDisableLatch_flg), VAEB_DriverDisableLatch_flg/1
  AEB Determination/3(VAEB_ForcedIdle_flg) -> VAEB_ForcedIdle_flg/1
  AEB Determination/1(VAEB_AEBActive_flg) -> VAEB_AEBActive_flg/1, [VAEB_AEBActive_flg]
  AEB Determination/2(VAEB_FCWActive_flg) -> VAEB_FCWActive_flg/1
  VDINR_SteerAngle_deg/1 -> Driver Disable/1(VDINR_SteerAngle_deg)
  VDINR_SteerAngleValid_flg/1 -> Driver Disable/2(VDINR_SteerAngleValid_flg)
  VDINR_HWAccelPedalPosn_pct/1 -> Driver Disable/3(VDINR_HWAccelPedalPosn_pct)
  VDINR_HWAccelPedalPosnValid_flg/1 -> Driver Disable/4(VDINR_HWAccelPedalPosnValid_flg)
  Driver Disable/1(VAEB_DriverDisable_flg) -> AEB Determination/1(VAEB_DriverDisable_flg), VAEB_DriverDisable_flg/1
  VDINR_VehSpd_kph/1 -> AEB Determination/4(VDINR_VehSpd_kph)

== system AEBMIL/AEB/model_info ==
  EmptySubsystem : Subsystem

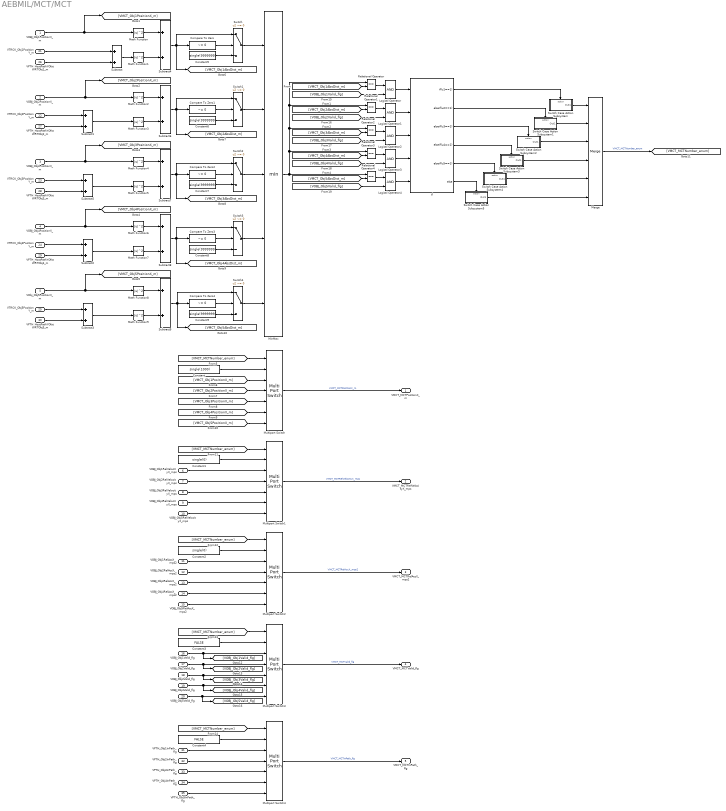
== system AEBMIL/MCT/MCT ==
  VOBJ_Obj1PositionX_m : Inport
  VOBJ_Obj2PositionX_m : Inport  Port=2
  VOBJ_Obj3PositionX_m : Inport  Port=3
  VOBJ_Obj4PositionX_m : Inport  Port=4
  VObj_Obj5PositionX_m : Inport  Port=5
  VOBJ_Obj1RelVelocityX_mps : Inport  Port=6
  VOBJ_Obj2RelVelocityX_mps : Inport  Port=7
  VOBJ_Obj3RelVelocityX_mps : Inport  Port=8
  VOBJ_Obj4RelVelocityX_mps : Inport  Port=9
  VOBJ_Obj5RelVelocityX_mps : Inport  Port=10
  VOBJ_Obj1RelAccX_mps2 : Inport  Port=11
  VOBJ_Obj2RelAccX_mps2 : Inport  Port=12
  VOBJ_Obj3RelAccX_mps2 : Inport  Port=13
  VOBJ_Obj4RelAccX_mps2 : Inport  Port=14
  VOBJ_Obj5RelAccX_mps2 : Inport  Port=15
  VOBJ_Obj1Valid_flg : Inport  Port=16
  VOBJ_Obj2Valid_flg : Inport  Port=17
  VOBJ_Obj3Valid_flg : Inport  Port=18
  VOBJ_Obj4Valid_flg : Inport  Port=19
  VOBJ_Obj5Valid_flg : Inport  Port=20
  VTRCK_Obj1PositionY_m : Inport  Port=21
  VTRCK_Obj2PositionY_m : Inport  Port=22
  VTRCK_Obj3PositionY_m : Inport  Port=23
  VTRCK_Obj4PositionY_m : Inport  Port=24
  VTRCK_Obj5PositionY_m : Inport  Port=25
  VPTH_HostPathYOfstWRTObj1_m : Inport  Port=26
  VPTH_HostPathYOfstWRTObj2_m : Inport  Port=27
  VPTH_HostPathYOfstWRTObj3_m : Inport  Port=28
  VPTH_HostPathYOfstWRTObj4_m : Inport  Port=29
  VPTH_HostPathYOfstWRTObj5_m : Inport  Port=30
  VPTH_Obj1InPath_flg : Inport  Port=31
  VPTH_Obj2InPath_flg : Inport  Port=32
  VPTH_Obj3InPath_flg : Inport  Port=33
  VPTH_Obj4InPath_flg : Inport  Port=34
  VPTH_Obj5InPath_flg : Inport  Port=35
  Compare To Zero{,1..4} (5 alike) : simulink/Logic and Bit Operations/Compare To Zero  relop=~=  OutDataTypeStr=boolean
  Constant : Constant  Value=single(1000)
  Constant1 : Constant  Value=single(0)
  Constant2 : Constant  Value=single(0)
  Constant3 : Constant  Value=FALSE
  Constant4 : Constant  Value=FALSE
  Constant{5..9} (5 alike) : Constant  Value=single(9999999)
  If : If  NumInputs=5  IfExpression=u1==1  ElseIfExpressions=u2==1,u3==1,u4==1,u5==1
  Logical Operator{,1..4} (5 alike) : Logic  AllPortsSameDT=off  OutDataTypeStr=boolean
  Math Function{,1..9} (10 alike) : Math  Operator=magnitude^2  SaturateOnIntegerOverflow=on
  Merge : Merge  Inputs=6
  MinMax : MinMax  Inputs=5
  Multiport Switch{,1..4} (5 alike) : MultiPortSwitch  DataPortOrder=Zero-based contiguous  Inputs=6
  Relational Operator{,1..4} (5 alike) : RelationalOperator  Operator===  OutDataTypeStr=boolean
  Subtract{,1..9} (10 alike) : Sum
  Switch{,1..4} (5 alike) : Switch  Criteria=u2 ~= 0
  Switch Case Action Subsystem : Subsystem  TreatAsAtomicUnit=on
  Switch Case Action Subsystem1 : Subsystem  TreatAsAtomicUnit=on
  Switch Case Action Subsystem2 : Subsystem  TreatAsAtomicUnit=on
  Switch Case Action Subsystem3 : Subsystem  TreatAsAtomicUnit=on
  Switch Case Action Subsystem4 : Subsystem  TreatAsAtomicUnit=on
  Switch Case Action Subsystem5 : Subsystem  TreatAsAtomicUnit=on
  VMCT_MCTPositionX_m : Outport
  VMCT_MCTRelVelocityX_mps : Outport  Port=2
  VMCT_MCTRelAccX_mps2 : Outport  Port=3
  VMCT_MCTValid_flg : Outport  Port=4
  VMCT_MCTInPath_flg : Outport  Port=5
  wires:
  Constant9/1 -> Switch4/3
  Switch4/1 -> MinMax/5
  Compare To Zero4/1 -> Switch4/2
  Subtract9/1 -> Switch4/1, [VMCT_Obj5AbsDist_m], Compare To Zero4/1
  Constant8/1 -> Switch3/3
  Switch3/1 -> MinMax/4
  Compare To Zero3/1 -> Switch3/2
  Subtract8/1 -> Compare To Zero3/1, Switch3/1, [VMCT_Obj4AbsDist_m]
  Constant7/1 -> Switch2/3
  Switch2/1 -> MinMax/3
  Compare To Zero2/1 -> Switch2/2
  Subtract7/1 -> Compare To Zero2/1, Switch2/1, [VMCT_Obj3AbsDist_m]
  Constant6/1 -> Switch1/3
  Switch1/1 -> MinMax/2
  Compare To Zero1/1 -> Switch1/2
  Subtract6/1 -> [VMCT_Obj2AbsDist_m], Compare To Zero1/1, Switch1/1
  Constant5/1 -> Switch/3
  Switch/1 -> MinMax/1
  Compare To Zero/1 -> Switch/2
  Constant4/1 -> Multiport Switch4/2
  Constant3/1 -> Multiport Switch3/2
  Constant2/1 -> Multiport Switch2/2
  Constant1/1 -> Multiport Switch1/2
  Constant/1 -> Multiport Switch/2
  Logical Operator4/1 -> If/5
  [VOBJ_Obj5Valid_flg] -> Logical Operator4/2
  [VOBJ_Obj4Valid_flg] -> Logical Operator3/2
  Logical Operator3/1 -> If/4
  [VOBJ_Obj3Valid_flg] -> Logical Operator2/2
  Logical Operator2/1 -> If/3
  [VOBJ_Obj2Valid_flg] -> Logical Operator1/2
  Logical Operator1/1 -> If/2
  [VOBJ_Obj1Valid_flg] -> Logical Operator/2
  Logical Operator/1 -> If/1
  Relational Operator/1 -> Logical Operator/1
  VOBJ_Obj5Valid_flg/1 -> Multiport Switch3/7, [VOBJ_Obj5Valid_flg]
  VOBJ_Obj4Valid_flg/1 -> [VOBJ_Obj4Valid_flg], Multiport Switch3/6
  VOBJ_Obj3Valid_flg/1 -> [VOBJ_Obj3Valid_flg], Multiport Switch3/5
  VOBJ_Obj2Valid_flg/1 -> Multiport Switch3/4, [VOBJ_Obj2Valid_flg]
  VPTH_Obj2InPath_flg/1 -> Multiport Switch4/4
  VPTH_Obj4InPath_flg/1 -> Multiport Switch4/6
  VPTH_Obj5InPath_flg/1 -> Multiport Switch4/7
  VPTH_Obj3InPath_flg/1 -> Multiport Switch4/5
  Multiport Switch4/1 -> VMCT_MCTInPath_flg/1  "VMCT_MCTInPath_flg"
  [VMCT_MCTNumber_enum] -> Multiport Switch4/1
  VPTH_Obj1InPath_flg/1 -> Multiport Switch4/3
  VOBJ_Obj1Valid_flg/1 -> [VOBJ_Obj1Valid_flg], Multiport Switch3/3
  [VMCT_MCTNumber_enum] -> Multiport Switch3/1
  VOBJ_Obj1RelAccX_mps2/1 -> Multiport Switch2/3
  VOBJ_Obj5RelAccX_mps2/1 -> Multiport Switch2/7
  VOBJ_Obj2RelAccX_mps2/1 -> Multiport Switch2/4
  VOBJ_Obj3RelAccX_mps2/1 -> Multiport Switch2/5
  VOBJ_Obj4RelAccX_mps2/1 -> Multiport Switch2/6
  [VMCT_MCTNumber_enum] -> Multiport Switch2/1
  VOBJ_Obj5RelVelocityX_mps/1 -> Multiport Switch1/7
  VOBJ_Obj4RelVelocityX_mps/1 -> Multiport Switch1/6
  VOBJ_Obj3RelVelocityX_mps/1 -> Multiport Switch1/5
  VOBJ_Obj2RelVelocityX_mps/1 -> Multiport Switch1/4
  VOBJ_Obj1RelVelocityX_mps/1 -> Multiport Switch1/3
  [VMCT_MCTNumber_enum] -> Multiport Switch1/1
  [VMCT_Obj1PositionX_m] -> Multiport Switch/3
  [VMCT_Obj5PositionX_m] -> Multiport Switch/7
  [VMCT_Obj4PositionX_m] -> Multiport Switch/6
  [VMCT_Obj2PositionX_m] -> Multiport Switch/4
  [VMCT_Obj3PositionX_m] -> Multiport Switch/5
  [VMCT_MCTNumber_enum] -> Multiport Switch/1
  Merge/1 -> [VMCT_MCTNumber_enum]  "VMCT_MCTNumber_enum"
  Switch Case Action Subsystem5/1(Out1) -> Merge/6
  Switch Case Action Subsystem4/1(Out1) -> Merge/5
  Switch Case Action Subsystem3/1(Out1) -> Merge/4
  Switch Case Action Subsystem2/1(Out1) -> Merge/3
  Switch Case Action Subsystem1/1(Out1) -> Merge/2
  Switch Case Action Subsystem/1(Out1) -> Merge/1
  If/6 -> Switch Case Action Subsystem5/Action
  If/5 -> Switch Case Action Subsystem4/Action
  If/4 -> Switch Case Action Subsystem3/Action
  If/3 -> Switch Case Action Subsystem2/Action
  If/2 -> Switch Case Action Subsystem1/Action
  If/1 -> Switch Case Action Subsystem/Action
  Relational Operator4/1 -> Logical Operator4/1
  Relational Operator1/1 -> Logical Operator1/1
  Relational Operator2/1 -> Logical Operator2/1
  Relational Operator3/1 -> Logical Operator3/1
  MinMax/1 -> Relational Operator3/1, Relational Operator2/1, Relational Operator1/1, Relational Operator/1, Relational Operator4/1
  [VMCT_Obj5AbsDist_m] -> Relational Operator4/2
  [VMCT_Obj4AbsDist_m] -> Relational Operator3/2
  [VMCT_Obj3AbsDist_m] -> Relational Operator2/2
  [VMCT_Obj2AbsDist_m] -> Relational Operator1/2
  [VMCT_Obj1AbsDist_m] -> Relational Operator/2
  Subtract4/1 -> [VMCT_Obj1AbsDist_m], Compare To Zero/1, Switch/1
  VObj_Obj5PositionX_m/1 -> [VMCT_Obj5PositionX_m], Math Function8/1
  Subtract3/1 -> Math Function9/1
  Math Function9/1 -> Subtract9/2
  Math Function8/1 -> Subtract9/1
  VTRCK_Obj5PositionY_m/1 -> Subtract3/1
  VPTH_HostPathYOfstWRTObj5_m/1 -> Subtract3/2
  VOBJ_Obj4PositionX_m/1 -> Math Function6/1, [VMCT_Obj4PositionX_m]
  Subtract2/1 -> Math Function7/1
  Math Function7/1 -> Subtract8/2
  Math Function6/1 -> Subtract8/1
  VTRCK_Obj4PositionY_m/1 -> Subtract2/1
  VPTH_HostPathYOfstWRTObj4_m/1 -> Subtract2/2
  VOBJ_Obj3PositionX_m/1 -> [VMCT_Obj3PositionX_m], Math Function4/1
  Subtract5/1 -> Math Function5/1
  Math Function5/1 -> Subtract7/2
  Math Function4/1 -> Subtract7/1
  VTRCK_Obj3PositionY_m/1 -> Subtract5/1
  VPTH_HostPathYOfstWRTObj3_m/1 -> Subtract5/2
  VOBJ_Obj2PositionX_m/1 -> Math Function2/1, [VMCT_Obj2PositionX_m]
  Subtract1/1 -> Math Function3/1
  Math Function3/1 -> Subtract6/2
  Math Function2/1 -> Subtract6/1
  Math Function1/1 -> Subtract4/2
  Math Function/1 -> Subtract4/1
  Subtract/1 -> Math Function1/1
  VTRCK_Obj2PositionY_m/1 -> Subtract1/1
  VPTH_HostPathYOfstWRTObj2_m/1 -> Subtract1/2
  VTRCK_Obj1PositionY_m/1 -> Subtract/1
  VPTH_HostPathYOfstWRTObj1_m/1 -> Subtract/2
  Multiport Switch3/1 -> VMCT_MCTValid_flg/1  "VMCT_MCTValid_flg"
  Multiport Switch2/1 -> VMCT_MCTRelAccX_mps2/1  "VMCT_MCTRelAccX_mps2"
  Multiport Switch1/1 -> VMCT_MCTRelVelocityX_mps/1  "VMCT_MCTRelVelocityX_mps"
  Multiport Switch/1 -> VMCT_MCTPositionX_m/1  "VMCT_MCTPositionX_m"
  VOBJ_Obj1PositionX_m/1 -> [VMCT_Obj1PositionX_m], Math Function/1

== system AEBMIL/MCT/model_info ==
  EmptySubsystem : Subsystem
